simulink model "fcaa"  (R2023a)
settings: Solver=VariableStepAuto  StartTime=0.0  StopTime=inf  RelTol=1e-3
settings Model: Creator=ardasengenc  LastModifiedBy=berkayozgur
settings HardwareCC: ProdBitPerLong=64  ProdHWDeviceType=Intel->x86-64 (Mac OS X)

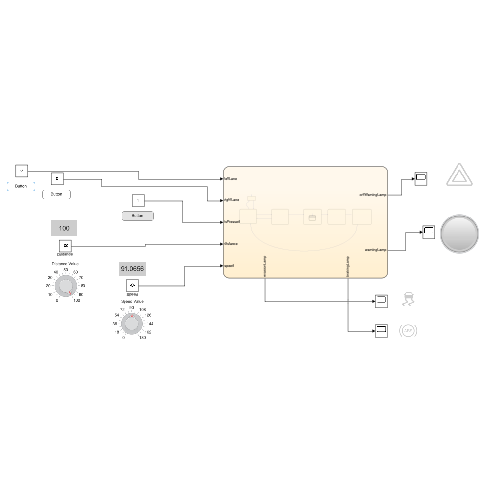
[thumbnail: Simulink's stored preview of the top-level diagram]
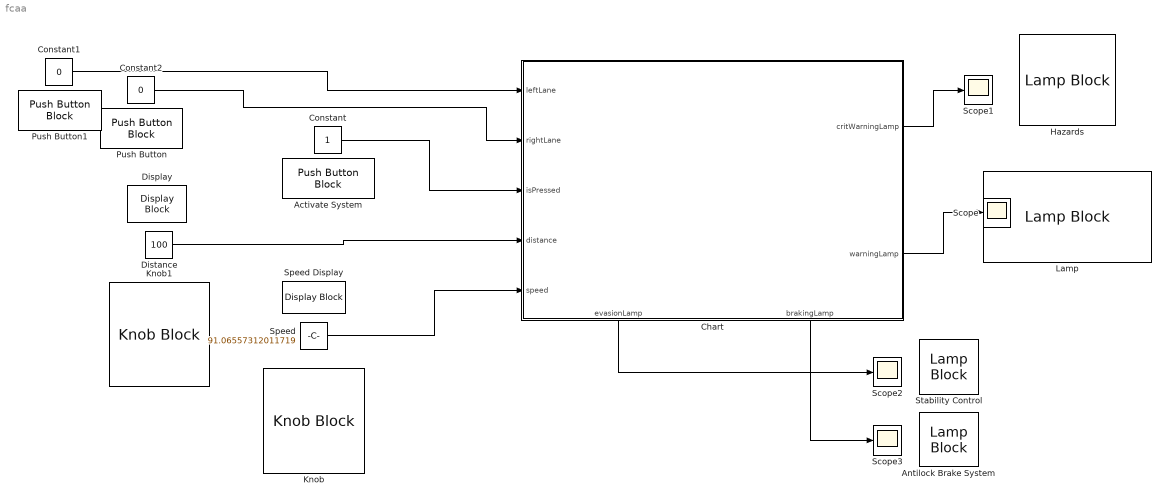
== system fcaa ==
  Activate System : PushButtonBlock  ButtonType=Latch  OffValue=0.000000
  Antilock Brake System : LampBlock  LabelPosition=Hide  Icon=AntilockBrakeSystem
  Chart : Stateflow chart  TreatAsAtomicUnit=on
      settings: PortSchema="{\"entries\":[{\"content\":{\"sides\":[{\"content\":{\"connectorIds\":[\"In1\",\"In2\",\"In3\",\"In4\",\"In5\"]},\"type\":\"ConnectorPlacement.EquallySpacedRectSide\",\"uuid\":\"bb82dbc6-565a-48e2-a270-6c5f1a85c48d\"},{\"content\":{\"connectorIds\":[\"Out3\",\"Out4\"],\"side\":\"RIGHT\"},\"type\":\"ConnectorPlacement.EquallySpacedRectSide\",\"uuid\":\"af29e780-d849-487b-8c17-f69bc4a7dc2c\"},{\"content\":{\"side\":\"TOP\"},\"type\":\"ConnectorPlacement.EquallySpacedRectSide\",\"uuid\":\"845e8555-5cd7-4c3e-b7e7-0a73fd5833bd\"},{\"content\":{\"connectorIds\":[\"Out1\",\"Out2\"],\"side\":\"BOTTOM\"},\"type\":\"ConnectorPlacement.EquallySpacedRectSide\",\"uuid\":\"0ad0b571-2219-4485-aa03-c58f1d1e49be\"}]},\"type\":\"ConnectorPlacement.EquallySpacedConnector\",\"uuid\":\"084560d0-55a7-4a41-8d3d-6682b36806cc\"}],\"packageUris\":[\"http://schema.mathworks.com/mf0/Connector/R2020b\"],\"version\":\"1.0\"}"
  Constant : Constant
  Constant1 : Constant  Value=0
  Constant2 : Constant  Value=0
  Display : DisplayBlock  LabelPosition=Hide  Transparency=1
  Distance : Constant  Value=100
  Hazards : LampBlock  LabelPosition=Hide  Icon=Hazards
  Knob : KnobBlock  ScaleMax=180
  Knob1 : KnobBlock
  Lamp : LampBlock  LabelPosition=Hide
  Push Button : PushButtonBlock  ButtonType=Latch  OffValue=0.000000
  Push Button1 : PushButtonBlock  ButtonType=Latch  OffValue=0.000000
  Scope{,1..3} (4 alike) : Scope
  Speed : Constant  Value=91.06557312011719
  Speed Display : DisplayBlock  LabelPosition=Hide  Transparency=1
  Stability Control : LampBlock  LabelPosition=Hide  Icon=StabilityControl
  wires:
  Constant/1 -> Chart/3(isPressed)
  Speed/1 -> Chart/5(speed)
  Distance/1 -> Chart/4(distance)
  Chart/4(warningLamp) -> Scope/1
  Chart/3(critWarningLamp) -> Scope1/1
  Constant1/1 -> Chart/1(leftLane)
  Constant2/1 -> Chart/2(rightLane)
  Chart/1(evasionLamp) -> Scope2/1
  Chart/2(brakingLamp) -> Scope3/1

== stateflow chart fcaa/Chart ==
  state OffState
  state Standby
    warningLamp = 0;
    critWarningLamp = 0;
    breakingDist = (speed/10)*(speed/10);
  state Warning
    warningLamp = 1;
    breakingDist = (speed/10)*(speed/10);
    emergencyDist = breakingDist/2;
    brakingLamp = 0;
    evasionLamp = 0;
  state Decision
    critWarningLamp = 1;
    state DecisionTree
      state Start
        brakingLamp = 0;
        evasionLamp = 0;
      state Brake
        brakingLamp = 1;
      state Evasion
        evasionLamp = 1;
      (default) -> Start
      Start -> Brake [order 1] : [(leftLane + rightLane) == 0]
      Start -> Evasion [order 2] : [leftLane == 1 || rightLane == 1]
    (default) -> DecisionTree
  state Control
  state Completed
  (default) -> OffState
  Standby -> OffState [order 2] : [isPressed == 0]
  OffState -> Standby : [isPressed == 1 && speed > 10]
  Standby -> Warning [order 1] : [distance < breakingDist]
      | %hier wäre die normale Bremsung
  Warning -> Decision [order 2] : [distance < emergencyDist]
      | %Hier die Notfallbremsung
  Decision -> Control : [(evasionLamp + brakingLamp) > 0]
  Control -> Completed
  Warning -> Standby [order 1] : [distance > breakingDist]
  Completed -> Standby : [distance > (speed/2)]
  data: evasionLamp output; brakingLamp output; leftLane input; rightLane input; critWarningLamp output; isPressed input; distance input; speed input; warningLamp output; emergencyDist local; breakingDist local
